simulink model "dual500MHzPFB"  (Simulink 6.2)
settings: Solver=ode45  StartTime=0.0  StopTime=10000  RelTol=1e-3
libraries: xbsIndex_r3 x2070, casper_library x180, xps_library x12, gtkWave x5, gavrt_library x1
(part 20 of 20)

== system dual500MHzPFB/cfgspec/FFT_Subsystem/fft_wideband_real1/fft_biplex_real_4x0/biplex_core/fft_stage_7/butterfly_direct/twiddle ==
  a : Inport  Port=1  LatchInput=off
  b : Inport  Port=2  LatchInput=off
  sync : Inport  Port=3  LatchInput=off
  twiddle_general_3mult : casper_library/FFTs/Twiddle/twiddle_general_3mult  Coeffs="[1+0i           6.1232e-017-1i               0.70711-0.70711i        -0.70711-0.70711i         0.92388-0.38268i        -0.38268-0.92388i         0.38268-0.92388i        -0.92388-0.38268i         0.98079-0.19509i        -0.19509-0.98079i         0.55557-0.83147i        -0.83147-0.55557i         0.83147-0.55557i        -0.55557-0.83147i         0.19509-0.98079i        -0.98079-0.19509i         0.99518-0.098017i      -0.098017-0.99518i         0.63439-0.77301i        -0.77301-0.63439i         0.88192-0.4714i          -0.4714-0.88192i         0.29028-0.95694i        -0.95694-0.29028i         0.95694-0.29028i        -0.29028-0.95694i          0.4714-0.88192i        -0.88192-0.4714i          0.77301-0.63439i        -0.63439-0.77301i        0.098017-0.99518i        -0.99518-0.098017i         0.9988-0.049068i      -0.049068-0.9988i          0.67156-0.74095i        -0.74095-0.67156i         0.90399-0.42756i        -0.42756-0.90399i         0.33689-0.94154i        -0.94154-0.33689i         0.97003-0.24298i        -0.24298-0.97003i          0.5141-0.85773i        -0.85773-0.5141i          0.80321-0.5957i          -0.5957-0.80321i         0.14673-0.98918i        -0.98918-0.14673i         0.98918-0.14673i        -0.14673-0.98918i          0.5957-0.80321i        -0.80321-0.5957i          0.85773-0.5141i          -0.5141-0.85773i         0.24298-0.97003i        -0.97003-0.24298i         0.94154-0.33689i        -0.33689-0.94154i         0.42756-0.90399i        -0.90399-0.42756i         0.74095-0.67156i        -0.67156-0.74095i        0.049068-0.9988i          -0.9988-0.049068i   ]"  StepPeriod=1  BitWidth=18  add_latency=3  mult_latency=3  bram_latency=2
  a_re : Outport
  a_im : Outport  Port=2
  bw_re : Outport  Port=3
  bw_im : Outport  Port=4
  sync_out : Outport  Port=5
  wires:
  a/1 -> twiddle_general_3mult/1
  b/1 -> twiddle_general_3mult/2
  sync/1 -> twiddle_general_3mult/3
  twiddle_general_3mult/1 -> a_re/1
  twiddle_general_3mult/2 -> a_im/1
  twiddle_general_3mult/3 -> bw_re/1
  twiddle_general_3mult/4 -> bw_im/1
  twiddle_general_3mult/5 -> sync_out/1

== system dual500MHzPFB/cfgspec/FFT_Subsystem/fft_wideband_real1/fft_biplex_real_4x0/biplex_core/fft_stage_8/butterfly_direct/twiddle ==
  a : Inport  Port=1  LatchInput=off
  b : Inport  Port=2  LatchInput=off
  sync : Inport  Port=3  LatchInput=off
  twiddle_general_3mult : casper_library/FFTs/Twiddle/twiddle_general_3mult  Coeffs="[1+0i           6.1232e-017-1i               0.70711-0.70711i        -0.70711-0.70711i         0.92388-0.38268i        -0.38268-0.92388i         0.38268-0.92388i        -0.92388-0.38268i         0.98079-0.19509i        -0.19509-0.98079i         0.55557-0.83147i        -0.83147-0.55557i         0.83147-0.55557i        -0.55557-0.83147i         0.19509-0.98079i        -0.98079-0.19509i         0.99518-0.098017i      -0.098017-0.99518i         0.63439-0.77301i        -0.77301-0.63439i         0.88192-0.4714i          -0.4714-0.88192i         0.29028-0.95694i        -0.95694-0.29028i         0.95694-0.29028i        -0.29028-0.95694i          0.4714-0.88192i        -0.88192-0.4714i          0.77301-0.63439i        -0.63439-0.77301i        0.098017-0.99518i        -0.99518-0.098017i         0.9988-0.049068i      -0.049068-0.9988i          0.67156-0.74095i        -0.74095-0.67156i         0.90399-0.42756i        -0.42756-0.90399i         0.33689-0.94154i        -0.94154-0.33689i         0.97003-0.24298i        -0.24298-0.97003i          0.5141-0.85773i        -0.85773-0.5141i          0.80321-0.5957i          -0.5957-0.80321i         0.14673-0.98918i        -0.98918-0.14673i         0.98918-0.14673i        -0.14673-0.98918i          0.5957-0.80321i        -0.80321-0.5957i          0.85773-0.5141i          -0.5141-0.85773i         0.24298-0.97003i        -0.97003-0.24298i         0.94154-0.33689i        -0.33689-0.94154i         0.42756-0.90399i        -0.90399-0.42756i         0.74095-0.67156i        -0.67156-0.74095i        0.049068-0.9988i          -0.9988-0.049068i         0.9997-0.024541i      -0.024541-0.9997i          0.68954-0.72425i        -0.72425-0.68954i         0.91421-0.40524i        -0.40524-0.91421i          0.3599-0.93299i        -0.93299-0.3599i           0.9757-0.2191i          -0.2191-0.9757i            0.535-0.84485i        -0.84485-0.535i           0.81758-0.57581i        -0.57581-0.81758i         0.17096-0.98528i        -0.98528-0.17096i         0.99248-0.12241i        -0.12241-0.99248i         0.61523-0.78835i        -0.78835-0.61523i         0.87009-0.4929i          -0.4929-0.87009i         0.26671-0.96378i        -0.96378-0.26671i         0.94953-0.31368i        -0.31368-0.94953i         0.44961-0.89322i        -0.89322-0.44961i         0.75721-0.65317i        -0.65317-0.75721i        0.073565-0.99729i        -0.99729-0.073565i        0.99729-0.073565i      -0.073565-0.99729i         0.65317-0.75721i        -0.75721-0.65317i         0.89322-0.44961i        -0.44961-0.89322i         0.31368-0.94953i        -0.94953-0.31368i         0.96378-0.26671i        -0.26671-0.96378i          0.4929-0.87009i        -0.87009-0.4929i          0.78835-0.61523i        -0.61523-0.78835i         0.12241-0.99248i        -0.99248-0.12241i         0.98528-0.17096i        -0.17096-0.98528i         0.57581-0.81758i        -0.81758-0.57581i         0.84485-0.535i            -0.535-0.84485i          0.2191-0.9757i          -0.9757-0.2191i          0.93299-0.3599i          -0.3599-0.93299i         0.40524-0.91421i        -0.91421-0.40524i         0.72425-0.68954i        -0.68954-0.72425i        0.024541-0.9997i          -0.9997-0.024541i   ]"  StepPeriod=0  BitWidth=18  add_latency=3  mult_latency=3  bram_latency=2
  a_re : Outport
  a_im : Outport  Port=2
  bw_re : Outport  Port=3
  bw_im : Outport  Port=4
  sync_out : Outport  Port=5
  wires:
  a/1 -> twiddle_general_3mult/1
  b/1 -> twiddle_general_3mult/2
  sync/1 -> twiddle_general_3mult/3
  twiddle_general_3mult/1 -> a_re/1
  twiddle_general_3mult/2 -> a_im/1
  twiddle_general_3mult/3 -> bw_re/1
  twiddle_general_3mult/4 -> bw_im/1
  twiddle_general_3mult/5 -> sync_out/1
